simulink model "uncontrolled_dynamics"  (R2020b)
settings: Solver=VariableStepAuto  StartTime=0.0  StopTime=10.0  RelTol=1e-3
undefined symbols (not defined in the file): orbit, spacecraft
libraries: sadc_library x4
settings Model: Creator=loren  LastModifiedBy=loren

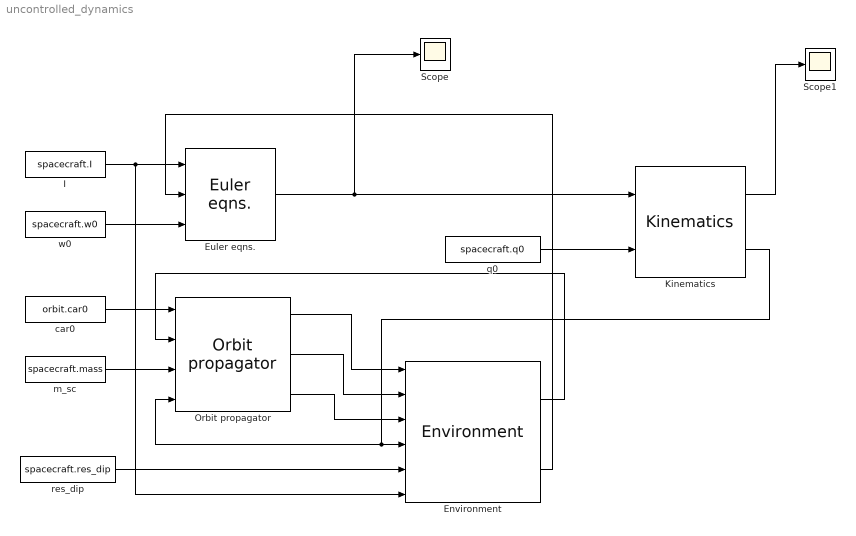
== system uncontrolled_dynamics ==
  Environment : sadc_library/Environment  SystemSampleTime=-1  VariantActivationTime=update diagram  Latency=0  AutoFrameSizeCalculation=off
  Euler eqns. : sadc_library/Euler eqns.  SystemSampleTime=-1  VariantActivationTime=update diagram  Latency=0  AutoFrameSizeCalculation=off
  I : Constant  Value=spacecraft.I
  Kinematics : sadc_library/Kinematics  SystemSampleTime=-1  VariantActivationTime=update diagram  Latency=0  AutoFrameSizeCalculation=off
  Orbit propagator : sadc_library/Orbit propagator  SystemSampleTime=-1  VariantActivationTime=update diagram  Latency=0  AutoFrameSizeCalculation=off
  Scope : Scope
  Scope1 : Scope
  car0 : Constant  Value=orbit.car0
  m_sc : Constant  Value=spacecraft.mass
  q0 : Constant  Value=spacecraft.q0
  res_dip : Constant  Value=spacecraft.res_dip
  w0 : Constant  Value=spacecraft.w0
  wires:
  I/1 -> Environment/6, Euler eqns./1
  w0/1 -> Euler eqns./3
  car0/1 -> Orbit propagator/1
  m_sc/1 -> Orbit propagator/3
  Orbit propagator/1 -> Environment/1
  Orbit propagator/2 -> Environment/2
  Orbit propagator/3 -> Environment/3
  res_dip/1 -> Environment/5
  Environment/1 -> Orbit propagator/2
  Environment/2 -> Euler eqns./2
  Euler eqns./1 -> Scope/1, Kinematics/1
  q0/1 -> Kinematics/2
  Kinematics/2 -> Orbit propagator/4, Environment/4
  Kinematics/1 -> Scope1/1
